simulink subsystem "model_3dof"  (R2025b)
settings: Solver=VariableStepAuto  StartTime=0.0  StopTime=10.0  RelTol=1e-3
values from neighbouring files (symbols this model uses):
  a = 13.06    [params.m]    (also in params_3dof.m = 0.0013; test.m = 0.0013)
  b = 0.0859    [params.m]    (also in params_3dof.m = 8.5908; test.m = 8.5908)
  d = 0.05    [params_1dof.m]    (also in params_3dof.m = 0.03)
  E = [ ... (first row only)    [params_3dof.m]    (also in test.m)
  g = 9.81    [params.m]    (also in params_1dof.m; params_3dof.m)
  guenther = 1.2    [params_3dof.m]
  I = diag([I_xx, I_yy, I_zz])    [params_3dof.m]
  m = 1.210    (= 1.21)    [params.m]    (also in params_1dof.m = 1.014; params_3dof.m = 1.014)
  p = [p_x, p_y, p_z]    [params.m]    (also in params_3dof.m = 0.2)
  T_delay_actor = 0    [params.m]    (also in params_3dof.m)
settings Model: Creator=schwmaxi  LastModifiedBy=schwmaxi

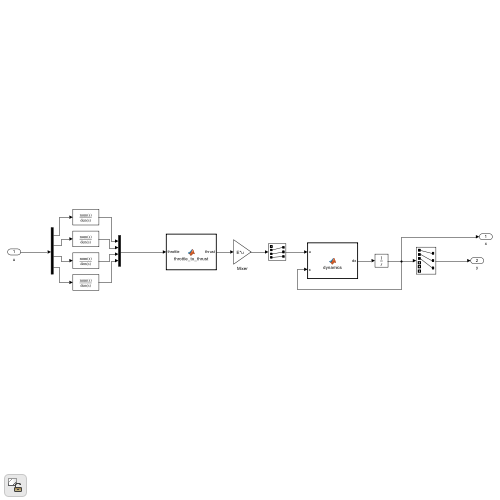
[thumbnail: Simulink's stored preview of the top-level diagram]
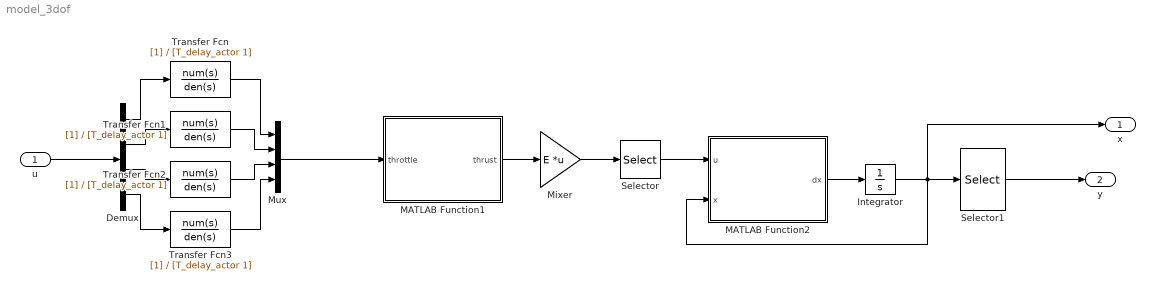
== system model_3dof ==
  u : Inport  OutDataTypeStr=double  PortDimensions=4  SampleTime=0
  Demux : Demux
  Integrator : Integrator
  MATLAB Function1 : MATLAB Function  TreatAsAtomicUnit=on
  MATLAB Function2 : MATLAB Function  TreatAsAtomicUnit=on
  Mixer : Gain  Gain=E  Multiplication=Matrix(K*u)
  Mux : Mux
  Selector : Selector  InputPortWidth=4  IndexOptions=Index vector (dialog)  Indices=[2 3 4]  OutputSizes=1
  Selector1 : Selector  InputPortWidth=6  IndexOptions=Index vector (dialog)  Indices=[1 2 3]  OutputSizes=1
  Transfer Fcn{,1..3} (4 alike) : TransferFcn  Denominator=[T_delay_actor 1]
  x : Outport  OutDataTypeStr=double  SampleTime=0
  y : Outport  Port=2  OutDataTypeStr=double  SampleTime=0
  wires:
  Selector/1 -> MATLAB Function2/1(u)
  MATLAB Function2/1(dx) -> Integrator/1
  Integrator/1 -> Selector1/1, MATLAB Function2/2(x), x/1
  Mixer/1 -> Selector/1
  MATLAB Function1/1(thrust) -> Mixer/1
  Transfer Fcn3/1 -> Mux/4
  Demux/2 -> Transfer Fcn1/1
  Transfer Fcn2/1 -> Mux/3
  Demux/4 -> Transfer Fcn3/1
  Demux/1 -> Transfer Fcn/1
  Transfer Fcn1/1 -> Mux/2
  Demux/3 -> Transfer Fcn2/1
  u/1 -> Demux/1
  Transfer Fcn/1 -> Mux/1
  Mux/1 -> MATLAB Function1/1(throttle)
  Selector1/1 -> y/1

== matlab function model_3dof/MATLAB Function1 ==
  data: thrust output; throttle input; a parameter; b parameter; guenther parameter
function thrust = throttle_to_thrust(throttle, a, b, guenther)
    thrust = guenther * a * (throttle - b).^2;
end

== matlab function model_3dof/MATLAB Function2 ==
  data: u input; x input; dx output; I parameter; p parameter; m parameter; g parameter; d parameter
function dx = dynamics(u, x, I, p, m, g, d)
    % I und p wird als Parameter Data übergeben, vgl. Symbols Pane

    phi = x(1);
    theta = x(2);

    omega = x(4:6);

    body_to_euler_rates = [
        1, sin(phi) * tan(theta), cos(phi)*tan(theta);
        0, cos(phi), -sin(phi);
        0, sin(phi) / cos(theta), cos(phi)/cos(theta);
    ];
    
    damping_moments = zeros(3, 1);
    damping_moments(1) = p * omega(1);

    angles_dot = body_to_euler_rates * omega(:);
    
    u(1) = u(1) + m * g * sin(phi) * cos(theta) * d;
    u(2) = u(2) + m * g * sin(theta) * d;

    omega_dot = I \ (u - damping_moments - cross(omega, I * omega));

    dx = [angles_dot; omega_dot];
end
